simulink model "fusion_des_travaux_bloc_NMPC_MATLAB_V2_TEST_AVEC_CAM"  (R2024b)
settings: Solver=ode1  StartTime=0.0  StopTime=inf  FixedStep=0.1  RelTol=1e-3  EnableMultiTasking=on
PostLoadFcn:
  | qlabs_setup
model workspace (MAT data in the model file):
  Sig : Simulink.Signal (value not decoded)
  downCamStepSize : Simulink.Parameter (value not decoded)
  lidarStepSize : Simulink.Parameter (value not decoded)
  mainStepSize : Simulink.Parameter (value not decoded)
  mode : Simulink.Parameter (value not decoded)
  realSenseStepSize : Simulink.Parameter (value not decoded)
values from neighbouring files (symbols this model uses):
  map = zeros(mapHeight*pointPerMeter, mapWidth*pointPerMeter)    [map_creator.m]    (also in map_creator_real.m)
  obstacles = [obstacles; coordinateX, coordinateY, rayon;]    [init.m]    (also in init1.m; init_V2.m; init_V3.m; map_creator.m = [)
  pointPerMeter = 50    [map_creator.m]    (also in map_creator_real.m)
  waypoints = [ ... (first row only)    [init.m]    (also in init1.m; init_V2.m; init_V3.m)
  x = input("Veuillez entrer la position x: ")    [map_creator_real.m]
symbols that are objects in the model workspace (value not decoded): downCamStepSize, lidarStepSize, mainStepSize, realSenseStepSize
undefined symbols (not defined in the file or in its folder): DiscIntNeverNeededParam, gcbh, JPEG, Point, qc_get_step_size, Video3D, video_display_show
libraries: quarc_library x27, simulink_extras x2, mpclib x1
(part 2 of 2)

== matlab function fusion_des_travaux_bloc_NMPC_MATLAB_V2_TEST_AVEC_CAM/MATLAB Function1 ==
  data: t input; X_ref output size=[3, 25]; obstacles input; waypoints input; is_final_approach output
function [X_ref, is_final_approach] = Traj_bezier_horizon(t, obstacles, waypoints)
    % Entrées : 
    %   t          : Temps de simulation actuel (secondes)
    %   obstacles  : Matrice des obstacles [x, y, rayon]
    %   waypoints  : Matrice des points de passage [x, y, theta]
    % Sorties : 
    %   X_ref            : Matrice [3 x Np] contenant les références futures [x; y; theta]
    %   kappa_actuel     : Scalaire de la courbure locale à l'instant t
    %   is_final_approach: Flag (0 ou 1) indiquant l'approche finale

    coder.extrinsic('plot', 'fill', 'quiver', 'figure', 'unwrap', 'warning');

    Ts = 0.1;   % Pas de temps 
    Np = 25;  

    X_ref             = zeros(3, Np);
    kappa_actuel      = 0;
    is_final_approach = 0;

    % Mémoire persistante avec types explicites pour le Coder
    persistent time_ref x_ref y_ref theta_ref kappa_ref initialized

    if isempty(initialized)
        initialized = int32(0);
        v_max = 0.5;
        omega_max = 2.0; 

        obstacles_rect   = [];
        n_points_per_seg = 1000;
        marge_securite   = 0.6;

        % typée double(0x1) pour que le Coder Simulink puisse inférer le type correctement
        x_total     = zeros(0, 1);
        y_total     = zeros(0, 1);
        theta_total = zeros(0, 1);
        kappa_total = zeros(0, 1);
        time_total  = zeros(0, 1);
        cumul_time  = 0;

        for seg = 1:(size(waypoints, 1) - 1)

            x_start = waypoints(seg,   1);  y_start = waypoints(seg,   2);  theta_start = waypoints(seg,   3);
            x_goal  = waypoints(seg+1, 1);  y_goal  = waypoints(seg+1, 2);  theta_goal  = waypoints(seg+1, 3);

            distance = sqrt((x_goal - x_start)^2 + (y_goal - y_start)^2);
            if distance < 1e-3
                warning('Traj_bezier_horizon: segment %d ignoré (distance < 1e-3).', seg);
                continue;
            end

            longueur_tangente = distance / 3;

            P0 = [x_start, y_start];
            P1 = P0 + longueur_tangente * [cos(theta_start), sin(theta_start)];
            P2 = [x_goal, y_goal] - longueur_tangente * [cos(theta_goal), sin(theta_goal)];
            P3 = [x_goal, y_goal];

            % Répulsion des points de contrôle vis-à-vis des obstacles circulaires
            for i = 1:size(obstacles, 1)
                obs_c = obstacles(i, 1:2);
                r_obs = obstacles(i, 3);

                if norm(P1 - obs_c) < r_obs + marge_securite + 0.5
                    dir = (P1 - obs_c) / norm(P1 - obs_c);
                    P1  = obs_c + dir * (r_obs + marge_securite + 0.2);
                end
                if norm(P2 - obs_c) < r_obs + marge_securite + 0.5
                    dir = (P2 - obs_c) / norm(P2 - obs_c);
                    P2  = obs_c + dir * (r_obs + marge_securite + 0.8);
                end
            end

            % Répulsion vis-à-vis des obstacles rectangulaires
            for i = 1:size(obstacles_rect, 1)
                xc  = obstacles_rect(i, 1);  yc  = obstacles_rect(i, 2);
                W   = obstacles_rect(i, 3);  H   = obstacles_rect(i, 4);
                ang = obstacles_rect(i, 5);
                R_mat       = [cos(ang), -sin(ang); sin(ang), cos(ang)];
                corners_loc = [-W/2, -H/2; W/2, -H/2; W/2, H/2; -W/2, H/2];
                corners_glob = (R_mat * corners_loc')' + [xc, yc];
                r_coin = 0.3;

                for j = 1:4
                    coin = corners_glob(j, :);
                    if norm(P1 - coin) < r_coin + marge_securite + 0.5
                        dir = (P1 - coin) / norm(P1 - coin);
                        P1  = coin + dir * (r_coin + marge_securite + 0.8);
                    end
                    if norm(P2 - coin) < r_coin + marge_securite + 0.5
                        dir = (P2 - coin) / norm(P2 - coin);
                        P2  = coin + dir * (r_coin + marge_securite + 0.8);
                    end
                end
            end

            % Génération de la courbe de Bézier cubique
            tt    = linspace(0, 1, n_points_per_seg)';
            x_seg = (1-tt).^3*P0(1) + 3*(1-tt).^2.*tt*P1(1) + 3*(1-tt).*tt.^2*P2(1) + tt.^3*P3(1);
            y_seg = (1-tt).^3*P0(2) + 3*(1-tt).^2.*tt*P1(2) + 3*(1-tt).*tt.^2*P2(2) + tt.^3*P3(2);

            dx  = gradient(x_seg);
            dy  = gradient(y_seg);
            ddx = gradient(dx);
            ddy = gradient(dy);

            theta_seg = atan2(dy, dx);
            kappa     = (dx.*ddy - dy.*ddx) ./ ((dx.^2 + dy.^2).^(3/2) + 1e-6);
            kappa(isnan(kappa)) = 0;

            % Profil de vitesse adaptatif (ralentissement dans les virages)
            v_seg = v_max * ones(size(kappa));
            for k = 1:length(kappa)
                if abs(kappa(k)) > 0.01
                    v_lim    = sqrt(3.0 / abs(kappa(k)));
                    v_seg(k) = min(v_seg(k), v_lim);
                end
            end
            v_seg = min(v_seg, v_max);

            % Conversion paramètre [0,1] → temps réel
            ds       = [0; sqrt(diff(x_seg).^2 + diff(y_seg).^2)];
            dt_seg   = ds ./ max(v_seg, 0.01);
            time_seg = cumsum(dt_seg) + cumul_time;

            if seg == 1
                x_total     = [x_total;     x_seg];     
                y_total     = [y_total;     y_seg];     
                theta_total = [theta_total; theta_seg]; 
                kappa_total = [kappa_total; kappa];     
                time_total  = [time_total;  time_seg]; 
            else
                x_total     = [x_total;     x_seg(2:end)];     
                y_total     = [y_total;     y_seg(2:end)];     
                theta_total = [theta_total; theta_seg(2:end)];
                kappa_total = [kappa_total; kappa(2:end)];     
                time_total  = [time_total;  time_seg(2:end)];  
            end

            cumul_time = time_total(end);
        end
        
        theta_total = unwrap(theta_total);

        % Stockage persistant
        time_ref  = time_total;
        x_ref     = x_total;
        y_ref     = y_total;
        theta_ref = theta_total;
        kappa_ref = kappa_total;

        % Tracé debug
        figure('Name', 'Trajectoire Bézier MPC', 'Position', [970 100 900 700]);
        hold on; grid on; axis equal;
        for i = 1:size(obstacles, 1)
            circle_x = obstacles(i,1) + obstacles(i,3) * cos(0:0.01:2*pi);
            circle_y = obstacles(i,2) + obstacles(i,3) * sin(0:0.01:2*pi);
            fill(circle_x, circle_y, [1 0.7 0.7], 'EdgeColor', 'r', 'LineWidth', 2);
        end
        plot(x_ref, y_ref, 'b-', 'LineWidth', 3);

        initialized = int32(1);

        % Au tout premier appel on retourne immédiatement les valeurs
        % par défaut déjà initialisées en tête (t=0 → pas encore de
        % trajectoire à interpoler de façon significative).

        return;
    end

    % ==========================================================
    % PHASE 2 : CALCUL DE LA MATRICE DE RÉFÉRENCE SUR L'HORIZON
    % ==========================================================

    % =========================================================
    % ARRÊT : on calcule la distance à l'arrivée en temps réel
    % à partir de la position estimée du robot (x_init passé en
    % entrée depuis le bloc MPC) mais ici on n'a pas x_init.
    % On utilise donc une double condition :
    %   - temporelle  : t > time_ref(end) - marge
    %   - ET spatiale : sera vérifiée côté MPC avec x_init réel
    % On réduit la marge temporelle à 0.5 s (au lieu de 2 s) pour
    % ne déclencher "final" qu'au dernier moment.
    % =========================================================
    dist_to_goal_ref = sqrt((interp1(time_ref, x_ref, min(t, time_ref(end)), 'linear') - x_ref(end))^2 + ...
                            (interp1(time_ref, y_ref, min(t, time_ref(end)), 'linear') - y_ref(end))^2);

    % if t > (time_ref(end) - 0.5) || dist_to_goal_ref < 0.3
    %     is_final_approach = 1;
    % else
    %     is_final_approach = 0;
    % end

    if t > time_ref(end)
        % Fin de trajectoire : on reste sur la dernière pose
        X_ref(1, :) = x_ref(end);
        X_ref(2, :) = y_ref(end);
        X_ref(3, :) = theta_ref(end);
        kappa_actuel = 0;
        is_final_approach = 1;
    else
        t_horizon        = t + (0:Np-1) * Ts;
        t_horizon_capped = min(t_horizon, time_ref(end));

        xr_vec     = interp1(time_ref, x_ref,     t_horizon_capped, 'linear');
        yr_vec     = interp1(time_ref, y_ref,     t_horizon_capped, 'linear');
        thetar_vec = interp1(time_ref, theta_ref, t_horizon_capped, 'linear');

        X_ref(1, :) = xr_vec;
        X_ref(2, :) = yr_vec;
        X_ref(3, :) = thetar_vec;
        is_final_approach = 0;
        kappa_actuel = interp1(time_ref, kappa_ref, t, 'spline');
    end
end

== matlab function fusion_des_travaux_bloc_NMPC_MATLAB_V2_TEST_AVEC_CAM/LiDAR analysis/Grid matching ==
  data: map input; x_rob input; y_rob input; ranges input; angles input; theta output double; pointPerMeter input
function theta = estimate_theta(map, x_rob, y_rob, ranges, angles, pointPerMeter)
    %#codegen
    % Note : x_rob et y_rob représentent ici la position du LiDAR, 
    % l'offset ayant été géré en amont dans le schéma Simulink.
    
    % --- Paramètres ---
    [mapRows, mapCols] = size(map);
    % On suppose que le centre de la matrice correspond aux coordonnées (0,0)
    center_row = mapRows / 2;
    center_col = mapCols / 2;
    
    % --- Filtrage des mesures LiDAR ---
    valid_idx = (ranges > 0) & (ranges < inf);
    r_valid = ranges(valid_idx);
    a_valid = angles(valid_idx);
    
    % --- Recherche de l'angle optimal (Scan Matching) ---
    % Test des angles de -pi à pi avec une résolution de 1 degré
    theta_search = -pi : (pi/180) : pi; 
    
    best_score = -1;
    best_theta = 0;
    
    % Boucle sur chaque angle possible
    for i = 1:length(theta_search)
        t = theta_search(i);
        
        % 1. Projection des points LiDAR dans le repère global
        % L'angle global du rayon est l'angle local du LiDAR + l'angle testé (t)
        x_pts = x_rob + r_valid .* cos(a_valid + t);
        y_pts = y_rob + r_valid .* sin(a_valid + t);
        
        % 2. Conversion des coordonnées monde (m) en indices de matrice (pixels)
        cols = round(center_col + (x_pts * pointPerMeter));
        rows = round(center_row - (y_pts * pointPerMeter)); 
        
        % 3. Filtrage de sécurité : on ignore les points hors de la carte
        in_bounds = (rows >= 1) & (rows <= mapRows) & (cols >= 1) & (cols <= mapCols);
        rows_in = rows(in_bounds);
        cols_in = cols(in_bounds);
        
        % 4. Calcul du score
        if isempty(rows_in)
            score = 0;
        else
            % Score = somme des "probabilités" d'obstacle sur la carte
            linear_indices = sub2ind([mapRows, mapCols], rows_in, cols_in);
            score = sum(map(linear_indices));
        end
        
        % 5. Mémorisation du meilleur angle
        if score > best_score
            best_score = score;
            best_theta = t;
        end
    end
    
    % Sortie finale
    theta = best_theta;
end

== matlab function fusion_des_travaux_bloc_NMPC_MATLAB_V2_TEST_AVEC_CAM/Subsystem/MATLAB Function3 ==
  data: depth_matrix input; dist_face_obstacle output; bord_gauche output; bord_droite output; alerte_securite output; img_debug output; rgb_matrix input
function [dist_face_obstacle, bord_gauche, bord_droite, alerte_securite, img_debug] = ...
         detecter_obstacles(depth_matrix, rgb_matrix)
% =========================================================================
% Bloc MATLAB Function - Détection d'obstacle par clustering de profondeur
% =========================================================================
% Principe : Dans la ROI centrale, on isole le cluster de pixels dont la
% profondeur est proche du minimum → face avant visible de l'obstacle.
%
% SORTIES :
%   dist_face_obstacle : distance minimale caméra → face avant obstacle (m)
%   bord_gauche        : colonne (px) du bord gauche dans l'image globale
%   bord_droite        : colonne (px) du bord droit dans l'image globale
%   alerte_securite    : true si obstacle détecté sous d_min_alerte (m)
%   img_debug          : matrice depth annotée (cadre ROI + bords obstacle)
%
% ROI centrale : lignes [40%–60%], colonnes [5%–95%] de l'image

    % =====================================================================
    % 1. PARAMÈTRES
    % =====================================================================
    Z_min             = cast(0.15,  'like', depth_matrix); % dist. min valide (m)
    Z_max             = cast(4.0,   'like', depth_matrix); % dist. max valide (m)
    d_min_alerte      = cast(0.4,   'like', depth_matrix); % seuil alerte sécurité (m)
    cluster_tolerance = cast(0.12,  'like', depth_matrix); % tolérance clustering face (m)
    min_cluster_ratio = 0.008; % fraction minimale de pixels ROI pour valider le cluster

    % =====================================================================
    % 2. INITIALISATIONS
    % =====================================================================
    [hauteur, largeur] = size(depth_matrix);

    dist_face_obstacle = Z_max;
    bord_gauche        = cast(0, 'like', depth_matrix);
    bord_droite        = cast(0, 'like', depth_matrix);
    alerte_securite    = false;
    img_debug          = depth_matrix;

    if hauteur < 10 || largeur < 10
        return;
    end

    % =====================================================================
    % 3. NETTOYAGE DE LA MATRICE DE PROFONDEUR
    % =====================================================================
    depth_clean = depth_matrix;
    masque_invalide = isnan(depth_clean)  | ...
                      isinf(depth_clean)  | ...
                      (depth_clean <= 0)  | ...
                      (depth_clean < Z_min) | ...
                      (depth_clean > Z_max);
    depth_clean(masque_invalide) = Z_max;

    % =====================================================================
    % 3.5. FILTRAGE PAR COULEUR (EXEMPLE : DÉTECTION DU ROUGE)
    % =====================================================================
    % Séparation des canaux RGB (l'image est en uint8, de 0 à 255)
    R = rgb_matrix(:,:,1);
    G = rgb_matrix(:,:,2);
    B = rgb_matrix(:,:,3);
    
    % Création d'un masque binaire : 1 si la couleur correspond, 0 sinon
    % faudra ajuster ces seuils selon l'éclairage de la salle en IRL
    seuil_rouge = 150;
    seuil_vert  = 100;
    seuil_bleu  = 100;
    masque_couleur = (R > seuil_rouge) & (G < seuil_vert) & (B < seuil_bleu);
    
    % On force la profondeur à Z_max pour tout ce qui N'EST PAS de la bonne couleur
    depth_clean(~masque_couleur) = Z_max;

    % =====================================================================
    % 4. ROI CENTRALE
    %    rC = [round(hauteur*0.4), round(hauteur*0.6)]
    %    cC = [round(largeur*0.05), round(largeur*0.95)]
    % =====================================================================
    r_start = max(1,       round(hauteur * 0.40));
    r_end   = min(hauteur, round(hauteur * 0.60));
    c_start = max(1,       round(largeur * 0.05));
    c_end   = min(largeur, round(largeur * 0.95));

    roi_C = depth_clean(r_start:r_end, c_start:c_end);
    [roi_h, roi_w] = size(roi_C);

    % =====================================================================
    % 5. CLUSTERING DE LA FACE AVANT DE L'OBSTACLE
    %
    % Inspiré du code MATLAB de clustering fourni :
    % On cherche le pixel le plus proche, puis on regroupe tous les pixels
    % dont la profondeur est dans [d_min, d_min + cluster_tolerance].
    % Ces pixels correspondent à la face plane de l'obstacle en face du robot.
    % =====================================================================

    % --- 5a. Masquer les pixels saturés à Z_max (pas d'obstacle)
    roi_valide = roi_C;
    roi_valide(roi_C >= Z_max) = NaN;

    % --- 5b. Distance minimale dans la ROI (obstacle le plus proche)
    d_min_roi = min(roi_valide(:));

    if isnan(d_min_roi) || isinf(d_min_roi)
        % Aucun obstacle valide dans la ROI → on quitte proprement
        img_debug = dessiner_cadre(img_debug, r_start, r_end, c_start, c_end);
        return;
    end

    % --- 5c. Masque de cluster : pixels appartenant à la face avant
    masque_cluster = (roi_C >= d_min_roi) & ...
                     (roi_C <= (d_min_roi + cluster_tolerance)) & ...
                     (roi_C  < Z_max);

    nb_pixels_cluster = sum(masque_cluster(:));
    nb_pixels_roi     = roi_h * roi_w;

    % Vérification : cluster assez grand pour être un obstacle réel
    if nb_pixels_cluster < round(min_cluster_ratio * nb_pixels_roi)
        img_debug = dessiner_cadre(img_debug, r_start, r_end, c_start, c_end);
        return;
    end

    % =====================================================================
    % 6. DISTANCE LA PLUS PROCHE (point de la face le plus près de la caméra)
    %
    % On prend le MINIMUM (et non la moyenne) pour avoir la distance réelle
    % entre la caméra et le point de surface le plus proche.
    % =====================================================================
    profondeurs_cluster = roi_C(masque_cluster);
    dist_face_obstacle  = cast(min(profondeurs_cluster), 'like', depth_matrix);

    % =====================================================================
    % 7. BORDS GAUCHE ET DROIT DE L'OBSTACLE
    %
    % On projette le masque sur l'axe horizontal.
    % Les colonnes occupées donnent l'emprise latérale de l'obstacle.
    % Conversion locale (dans la ROI) → globale (dans l'image entière).
    % =====================================================================
    cols_occupees = any(masque_cluster, 1); % vecteur 1×roi_w
    indices_cols  = find(cols_occupees);

    if ~isempty(indices_cols)
        bord_gauche = cast(c_start + indices_cols(1)   - 1, 'like', depth_matrix);
        bord_droite = cast(c_start + indices_cols(end) - 1, 'like', depth_matrix);
    end

    % =====================================================================
    % 8. ALERTE SÉCURITÉ — ROI CENTRALE UNIQUEMENT, seuil bas
    % =====================================================================
    if dist_face_obstacle <= d_min_alerte
        alerte_securite = true;
    end

    % =====================================================================
    % 9. TEMPS AVANT COLLISION (TTC) — COMMENTÉ
    %
    % Pour activer, passer la vitesse du robot en paramètre d'entrée.
    %
    % v_robot = 0.5;  % vitesse de déplacement du robot (m/s)
    % if v_robot > 0 && dist_face_obstacle < Z_max
    %     TTC = dist_face_obstacle / v_robot;
    %     % TTC en secondes. Si TTC < seuil_urgence → évitement immédiat.
    %     % Exemple : seuil_urgence = 1.5 s
    % else
    %     TTC = inf;
    % end
    %
    % NOTE : Pour plus de précision, utiliser la dérivée temporelle
    % de dist_face_obstacle entre deux frames :
    %   v_approche = (dist_prev - dist_face_obstacle) / dt;
    %   TTC = dist_face_obstacle / v_approche;  (si v_approche > 0)
    % =====================================================================

    % =====================================================================
    % 10. ESTIMATION ANGULAIRE DES BORDS (nécessite calibration caméra)
    %
    % Si tu connais la focale horizontale fx et le centre optique cx :
    %
    % fx = 462.0;  % pixels (valeur typique pour caméra QBot)
    % cx = largeur / 2;
    %
    % angle_bord_gauche = atan2d(double(bord_gauche) - cx, fx);  % degrés
    % angle_bord_droite = atan2d(double(bord_droite) - cx, fx);
    %
    % dist_laterale_gauche = dist_face_obstacle * tand(angle_bord_gauche);
    % dist_laterale_droite = dist_face_obstacle * tand(angle_bord_droite);
    % Ces distances en mètres indiquent l'offset latéral des bords.
    % =====================================================================

    % =====================================================================
    % 11. IMAGE DE DÉBOGAGE
    % =====================================================================
    % Cadre noir de la ROI
img_debug = dessiner_cadre(img_debug, r_start, r_end, c_start, c_end);

% --- BORDS DE L'OBSTACLE EN BLANC ---
% Valeur 10.0 = pixel blanc/brillant après normalisation (/10) pour le Video Viewer
    if bord_gauche > 0 && bord_droite > 0
        col_g = min(largeur, max(1, round(double(bord_gauche))));
        col_d = min(largeur, max(1, round(double(bord_droite))));
    
        % Ligne verticale blanche sur toute la hauteur de la ROI
        for r = r_start:r_end
            img_debug(r, col_g) = cast(10.0, 'like', depth_matrix); % bord gauche blanc
            img_debug(r, col_d) = cast(10.0, 'like', depth_matrix); % bord droit blanc
        end
    end

end % fin fonction principale

% =========================================================================
% SOUS-FONCTION : Dessin du cadre de la ROI
% =========================================================================
function img = dessiner_cadre(img, r_start, r_end, c_start, c_end)
    img(r_start:r_end, c_start) = 0;  % bord gauche ROI (noir)
    img(r_start:r_end, c_end)   = 0;  % bord droit ROI
    img(r_start, c_start:c_end) = 0;  % bord haut ROI
    img(r_end,   c_start:c_end) = 0;  % bord bas ROI
end

== matlab function fusion_des_travaux_bloc_NMPC_MATLAB_V2_TEST_AVEC_CAM/LiDAR analysis/Lidar & Localization/MATLAB Function ==
  data: lidar_position input; ranges input; ranges_c output; angles input; angles_c output
function [ranges_c,angles_c] = correct_lidar(lidar_position, ranges,angles)

x = ranges.*cos(angles) + lidar_position(1);
y = ranges.*sin(angles) + lidar_position(2);

ranges_c = sqrt(x.^2 + y.^2);
angles_c = atan2(y, x);

end

== matlab function fusion_des_travaux_bloc_NMPC_MATLAB_V2_TEST_AVEC_CAM/Extended Kalman filter ancien/MATLAB Function ==
  data: v input; X_pred output; w input; xk input; yk input; thetak input; P input; Y_pred output; theta_pred output; P_pred output
function [X_pred, Y_pred, theta_pred, P_pred] = prediction(v, w, xk, yk, thetak, P)
    Ts = 0.01;
    
    % Vecteur d'état actuel
    X = [xk; yk; thetak];
   
    % 1. MODÈLE D'ÉTAT (Cinématique du QBot)
    % On calcule la prédiction basée sur les vitesses v (linéaire) et w (angulaire)
    X_next = X + [v * cos(thetak) * Ts;
                  v * sin(thetak) * Ts;
                  w * Ts];
    
    % Extraction des sorties
    X_pred     = X_next(1);
    Y_pred     = X_next(2);
    % theta_pred = atan2(sin(X_next(3)), cos(X_next(3))); % Normalisation d'angle (-pi à pi)
    theta_pred =X_next(3);

    % 2. LINÉARISATION (Calcul de la Jacobienne F)
    % f est la dérivée de l'équation d'état par rapport à x, y et theta
    F = [1, 0, -v * Ts * sin(thetak);
         0, 1,  v * Ts *cos(thetak);
         0, 0,  1];

    % 3. BRUIT DE MODÈLE (Matrice Q)
    % Plus ces valeurs sont élevées, moins on fait confiance au modèle théorique
    % À ajuster
    q_x = 0.00001; %0.001
    q_y = 0.00001;%0.001
    q_theta = 0.00002;%0.002
    Q = diag([q_x, q_y, q_theta]);

    % 4. PRÉDICTION DE LA COVARIANCE
    % On propage l'incertitude P_pred = F*P*F' + Q
    P_pred = F * P * F' + Q;
end

== matlab function fusion_des_travaux_bloc_NMPC_MATLAB_V2_TEST_AVEC_CAM/Extended Kalman filter ancien/MATLAB Function1 ==
  data: X_pred input; X_est output; Y_pred input; theta_pred input; X_lidar input; Y_lidar input; theta_lidar input; P_pred input; Y_est output; theta_est output; P_est output
function [X_est, Y_est, theta_est, P_est] = update(X_pred, Y_pred, theta_pred, X_lidar, Y_lidar, theta_lidar, P_pred)
    % 1. VECTEURS D'ÉTAT ET DE MESURE
    x_p = [X_pred; Y_pred; theta_pred];
    z = [X_lidar; Y_lidar; theta_lidar];

    % 2. MODÈLE D'OBSERVATION (H)
    % Puisque le LIDAR mesure directement x, y et theta, H est l'identité
    H = eye(3);

    % 3. MATRICE DE BRUIT DE MESURE (R)
    % Plus ces valeurs sont faibles, plus le filtre fera confiance au LIDAR
    % (À ajuster selon la précision du LIDAR)
    r_dist = 0.00005; % Incertitude en mètres 0.05
    r_ang  = 0.00002; % Incertitude en radians0.02
    R = diag([r_dist, r_dist, r_ang]);

    % 4. CALCUL DU GAIN DE KALMAN (K)
    % S est la covariance de l'innovation
    S = H * P_pred * H' + R;
    K = P_pred * H' / S;

    % 5. CALCUL DE L'Erreur entre LIDAR et Prédiction
    innovation = z - (H * x_p);

    %Normalisation de l'erreur d'angle
    % Empêche le filtre de paniquer si le LIDAR dit 179° et le modèle 181° (-179°)
    innovation(3) = atan2(sin(innovation(3)), cos(innovation(3)));

    % 6. MISE À JOUR DE L'ÉTAT ET DE LA COVARIANCE
    x_corrected = x_p + K * innovation;
    P_corrected = (eye(3) - K * H) * P_pred;

    % 7. ASSIGNATION DES SORTIES
    X_est = x_corrected(1);
    Y_est = x_corrected(2);
    % theta_est = atan2(sin(x_corrected(3)), cos(x_corrected(3)));
    theta_est = x_corrected(3);
    P_est = P_corrected;
end

== matlab function fusion_des_travaux_bloc_NMPC_MATLAB_V2_TEST_AVEC_CAM/Extended Kalman filter1/MATLAB Function ==
  data: v input; X_pred output; w input; xk input; yk input; thetak input; P input; Y_pred output; theta_pred output; P_pred output
function [X_pred, Y_pred, theta_pred, P_pred] = prediction(v, w, xk, yk, thetak, P)
    Ts = 0.01;
    
    % Vecteur d'état actuel
    X = [xk; yk; thetak];
   
    % 1. MODÈLE D'ÉTAT (Cinématique du QBot)
    % On calcule la prédiction basée sur les vitesses v (linéaire) et w (angulaire)
    X_next = X + [v * cos(thetak) * Ts;
                  v * sin(thetak) * Ts;
                  w * Ts];
    
    % Extraction des sorties
    X_pred     = X_next(1);
    Y_pred     = X_next(2);
    % theta_pred = atan2(sin(X_next(3)), cos(X_next(3))); % Normalisation d'angle (-pi à pi)
    theta_pred =X_next(3);

    % 2. LINÉARISATION (Calcul de la Jacobienne F)
    % f est la dérivée de l'équation d'état par rapport à x, y et theta
    F = [1, 0, -v * Ts * sin(thetak);
         0, 1,  v * Ts *cos(thetak);
         0, 0,  1];

    % 3. BRUIT DE MODÈLE (Matrice Q)
    % Plus ces valeurs sont élevées, moins on fait confiance au modèle théorique
    % À ajuster
    q_x = 0.00001; %0.001
    q_y = 0.00001;%0.001
    q_theta = 0.00002;%0.002
    Q = diag([q_x, q_y, q_theta]);

    % 4. PRÉDICTION DE LA COVARIANCE
    % On propage l'incertitude P_pred = F*P*F' + Q
    P_pred = F * P * F' + Q;
end
